simulink model "butterworth_mdl"  (Simulink 7.6)
settings: Solver=ode45  StartTime=0.0  StopTime=0.25  RelTol=1e-3
values from neighbouring files (symbols this model uses):
  dt = 1/fs    (= 0.0025)    [butterworth.m]
undefined symbols (not defined in the file or in its folder): a, b
settings Model: Creator=gareths  LastModifiedBy=gareths

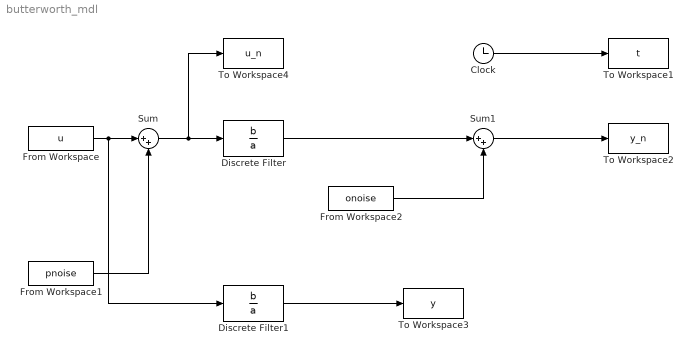
== system butterworth_mdl ==
  Clock : Clock
      settings: Decimation=10
  Discrete Filter : DiscreteFilter  Numerator=b  Denominator=a  SampleTime=dt
  Discrete Filter1 : DiscreteFilter  Numerator=b  Denominator=a  SampleTime=dt
  From Workspace : FromWorkspace  VariableName=u  SampleTime=0
  From Workspace1 : FromWorkspace  VariableName=pnoise  SampleTime=0
  From Workspace2 : FromWorkspace  VariableName=onoise  SampleTime=0
  Sum : Sum  Inputs=|++
  Sum1 : Sum  Inputs=|++
  To Workspace1 : ToWorkspace  VariableName=t  SampleTime=-1  SaveFormat=Array
  To Workspace2 : ToWorkspace  VariableName=y_n  SampleTime=-1  SaveFormat=Array
  To Workspace3 : ToWorkspace  VariableName=y  SampleTime=-1  SaveFormat=Array
  To Workspace4 : ToWorkspace  VariableName=u_n  SampleTime=-1  SaveFormat=Array
  wires:
  Clock/1 -> To Workspace1/1
  From Workspace/1 -> Sum/1, Discrete Filter1/1
  Sum/1 -> Discrete Filter/1, To Workspace4/1
  Discrete Filter/1 -> Sum1/1
  Sum1/1 -> To Workspace2/1
  Discrete Filter1/1 -> To Workspace3/1
  From Workspace2/1 -> Sum1/2
  From Workspace1/1 -> Sum/2
